simulink model "robot_capteur_etu"  (R2021a)
settings: Solver=VariableStepAuto  StartTime=0.0  StopTime=10.0  RelTol=1e-3
values from neighbouring files (symbols this model uses):
  K = -place(A,B,poles)    [matrices.m]    (also in simu_robot_etu.m = [0.6700 19.9055 1.0747 1.9614])
  ue = 0    [simu_robot_etu.m]
  x0 = [0 pi/10 0 0]    [simu_robot_etu.m]
  xe = [0 0 0 0]'    [simu_robot_etu.m]
settings Model: Creator=ysaoudi  LastModifiedBy=ialouane
settings SolverCC: AlgebraicLoopSolver=TrustRegion
settings DebuggingCC: SFMachineParentedDataDiag=warning
settings SFSimCC: CustomCodeUndefinedFunction=UseInterfaceOnly

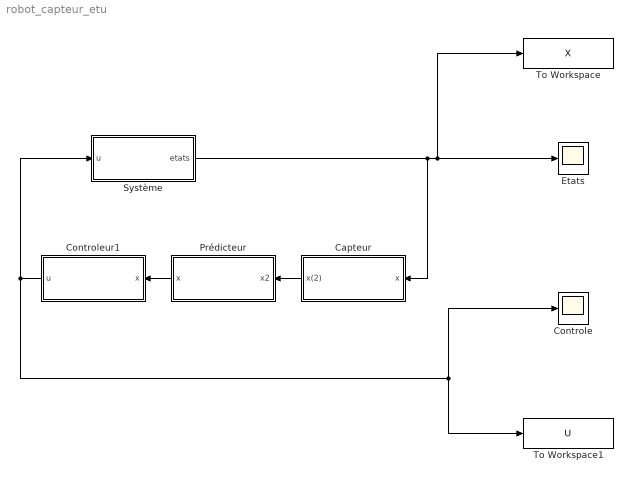
== system robot_capteur_etu ==
  Capteur : Subsystem
  Controle : Scope
  Controleur1 : Subsystem
  Etats : Scope
  Prédicteur : Subsystem
  Système : Subsystem
  To Workspace : ToWorkspace  VariableName=X  SaveFormat=Timeseries  SampleTime=-1
  To Workspace1 : ToWorkspace  VariableName=U  SaveFormat=Timeseries  SampleTime=-1
  wires:
  Capteur/1(x(2)) -> Prédicteur/1(x2)
  Système/1(etats) -> Capteur/1(x), To Workspace/1, Etats/1
  Controleur1/1(u) -> Système/1(u), To Workspace1/1, Controle/1
  Prédicteur/1(x) -> Controleur1/1(x)

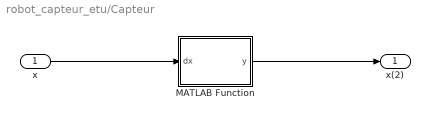
== system robot_capteur_etu/Capteur ==
  x : Inport
  MATLAB Function : MATLAB Function  TreatAsAtomicUnit=on
  x(2) : Outport
  wires:
  x/1 -> MATLAB Function/1(dx)
  MATLAB Function/1(y) -> x(2)/1

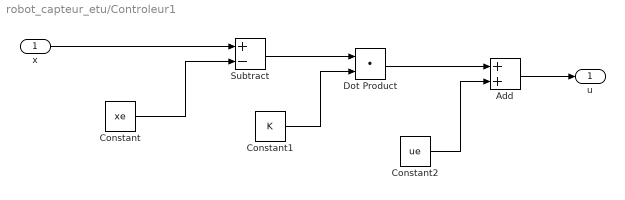
== system robot_capteur_etu/Controleur1 ==
  x : Inport
  Add : Sum
  Constant : Constant  Value=xe
  Constant1 : Constant  Value=K  VectorParams1D=off
  Constant2 : Constant  Value=ue
  Dot Product : DotProduct  InputSameDT=on  OutDataTypeStr=Inherit: Inherit via internal rule
  Subtract : Sum  Inputs=+-
  u : Outport
  wires:
  Add/1 -> u/1
  Constant2/1 -> Add/2
  Dot Product/1 -> Add/1
  Constant1/1 -> Dot Product/2
  Subtract/1 -> Dot Product/1
  Constant/1 -> Subtract/2
  x/1 -> Subtract/1

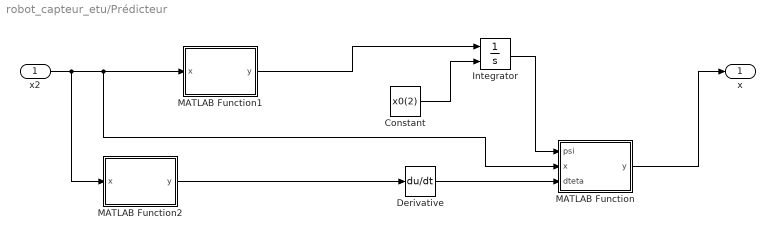
== system robot_capteur_etu/Prédicteur ==
  x2 : Inport
  Constant : Constant  Value=x0(2)
  Derivative : Derivative
  Integrator : Integrator  InitialConditionSource=external
  MATLAB Function : MATLAB Function  TreatAsAtomicUnit=on
  MATLAB Function1 : MATLAB Function  TreatAsAtomicUnit=on
  MATLAB Function2 : MATLAB Function  TreatAsAtomicUnit=on
  x : Outport
  wires:
  Constant/1 -> Integrator/2
  MATLAB Function/1(y) -> x/1
  x2/1 -> MATLAB Function2/1(x), MATLAB Function/2(x), MATLAB Function1/1(x)
  MATLAB Function1/1(y) -> Integrator/1
  Integrator/1 -> MATLAB Function/1(psi)
  Derivative/1 -> MATLAB Function/3(dteta)
  MATLAB Function2/1(y) -> Derivative/1

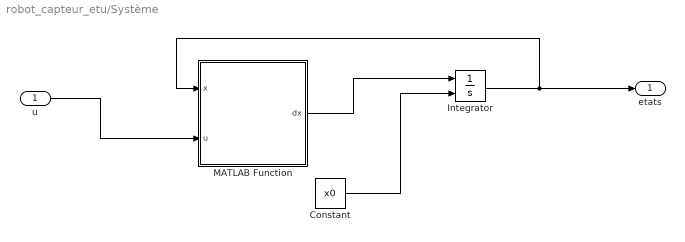
== system robot_capteur_etu/Système ==
  u : Inport
  Constant : Constant  Value=x0
  Integrator : Integrator  InitialConditionSource=external
  MATLAB Function : MATLAB Function  TreatAsAtomicUnit=on
  etats : Outport
  wires:
  u/1 -> MATLAB Function/2(u)
  MATLAB Function/1(dx) -> Integrator/1
  Constant/1 -> Integrator/2
  Integrator/1 -> MATLAB Function/1(x), etats/1

== matlab function robot_capteur_etu/Prédicteur/MATLAB Function1 ==
  data: x input; y output
function y = fcn(x)
y=x(2);
end

== matlab function robot_capteur_etu/Système/MATLAB Function ==
  data: x input; u input; dx output
function dx = fcn( x, u)
dx = fonction(x,u);
end

== matlab function robot_capteur_etu/Capteur/MATLAB Function ==
  data: dx input; y output
function y = fcn(dx)
y = [dx(1), dx(4)];
end

== matlab function robot_capteur_etu/Prédicteur/MATLAB Function ==
  data: psi input; x input; y output; dteta input
function y = fcn(psi,x,dteta)
y=[x(1);psi;dteta;x(2)];
end

== matlab function robot_capteur_etu/Prédicteur/MATLAB Function2 ==
  data: x input; y output
function y = fcn(x)
y = x(1);
end
